simulink model "Ex1_Arithmetic_operations"  (R2018b)
settings: Solver=VariableStepAuto  StartTime=0.0  StopTime=10.0  RelTol=1e-3
settings Model: Creator=sulaymon.eshkabilov  LastModifiedBy=sulaymon.eshkabilov

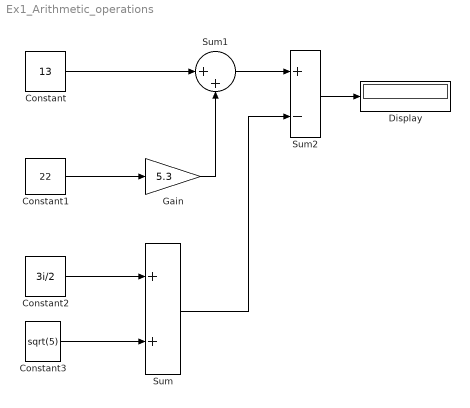
== system Ex1_Arithmetic_operations ==
  Constant : Constant  Value=13
  Constant1 : Constant  Value=22
  Constant2 : Constant  Value=3i/2
  Constant3 : Constant  Value=sqrt(5)
  Display : Display
  Gain : Gain  Gain=5.3
  Sum : Sum
  Sum1 : Sum  Inputs=|++
  Sum2 : Sum  Inputs=+-
  wires:
  Constant1/1 -> Gain/1
  Gain/1 -> Sum1/2
  Constant/1 -> Sum1/1
  Sum1/1 -> Sum2/1
  Constant2/1 -> Sum/1
  Constant3/1 -> Sum/2
  Sum/1 -> Sum2/2
  Sum2/1 -> Display/1
